simulink model "steppidsupport"  (Simulink 10.0)
settings: Solver=ode45  StartTime=0.0  StopTime=29.9132  FixedStep=0.005  RelTol=1e-5  EnableMultiTasking=on
settings Model: Creator=root  LastModifiedBy=bhisma
settings DataIOCC: LimitDataPoints=on  SignalLoggingSaveFormat=ModelDataLogs  SaveOutput=off  SaveTime=off  SignalLoggingName=sigsOut
settings OptimizationCC: LifeSpan=auto
settings DebuggingCC: SaveWithParameterizedLinksMsg=none  SignalResolutionControl=TryResolveAllWithWarning  MultiTaskDSMMsg=warning  MultiTaskCondExecSysMsg=none  SFUnexpectedBacktrackingDiag=error  SFNoUnconditionalDefaultTransitionDiag=error  SFExecutionAtInitializationDiag=warning  ArithmeticOperatorsInVariantConditions=error
settings HardwareCC: TargetUnknown=on
settings SFSimCC: SimUseLocalCustomCode=on  CustomCodeUndefinedFunction=FilterOut
settings RTWCC: RTWUseLocalCustomCode=on
settings CodeAppCC: StateflowObjectComments=off
settings GRTTargetCC: TargetLangStandard=C99 (ISO)

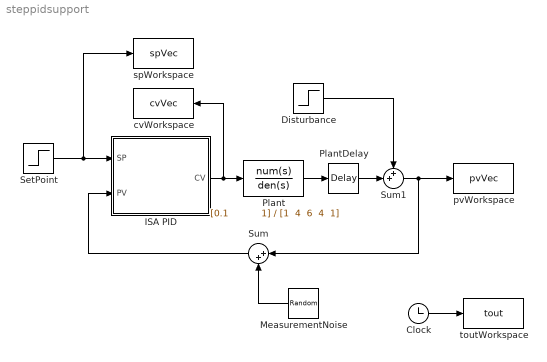
== system steppidsupport ==
  Clock : Clock
  Disturbance : Step  Time=19.9422  After=0.1  SampleTime=0
  ISA PID : Subsystem  mask{uaw=[-5 5], Ts=0.019995, As=1, histLevel=0}
      mask prompts: uaw "Antiwindup saturation ([umin,umax])"; Ts "Sample time (Ts)"; As "Amplitude of the identifcation step or relay (A)"; histLevel "Histeresys of the relay"
      mask init:
      | umin = uaw(1);
      | umax = uaw(2);
      mask Display: disp('ISA PID')
  MeasurementNoise : RandomNumber  Variance=0  SampleTime=0
  Plant : TransferFcn  Numerator="[0.1           1]"  Denominator="[1  4  6  4  1]"
  PlantDelay : TransportDelay  DelayTime=0.75
  SetPoint : Step  Time=0  SampleTime=0
  Sum : Sum  Inputs=|++  SaturateOnIntegerOverflow=on  InputSameDT=on  OutDataTypeStr=Inherit: Same as first input
  Sum1 : Sum  Inputs=++|  SaturateOnIntegerOverflow=on  InputSameDT=on  OutDataTypeStr=Inherit: Same as first input
  cvWorkspace : ToWorkspace  VariableName=cvVec  SampleTime=0.019995
  pvWorkspace : ToWorkspace  VariableName=pvVec  SampleTime=0.019995
  spWorkspace : ToWorkspace  VariableName=spVec  SampleTime=0.019995
  toutWorkspace : ToWorkspace  VariableName=tout  SampleTime=0.019995
  wires:
  SetPoint/1 -> spWorkspace/1, ISA PID/1(SP)
  ISA PID/1(CV) -> cvWorkspace/1, Plant/1
  MeasurementNoise/1 -> Sum/2
  Sum/1 -> ISA PID/2(PV)
  Clock/1 -> toutWorkspace/1
  Sum1/1 -> pvWorkspace/1, Sum/1
  Disturbance/1 -> Sum1/1
  Plant/1 -> PlantDelay/1
  PlantDelay/1 -> Sum1/2

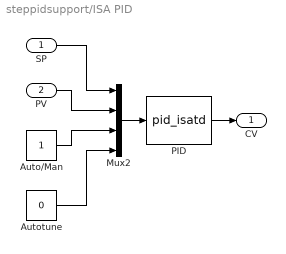
== system steppidsupport/ISA PID ==
  SP : Inport
  PV : Inport  Port=2
  Auto/Man : Constant
  Autotune : Constant  Value=0
  Mux2 : Mux
  PID : S-Function  FunctionName=pid_isatd  Parameters=Ts,umin,umax,As,histLevel  SFunctionDeploymentMode=off  EnableBusSupport=off
  CV : Outport
  wires:
  SP/1 -> Mux2/1
  PV/1 -> Mux2/2
  PID/1 -> CV/1
  Mux2/1 -> PID/1
  Auto/Man/1 -> Mux2/3
  Autotune/1 -> Mux2/4
